simulink library "SkywardBLIMP_back"  (R2015a)
settings: Solver=ode45  StartTime=0.0  StopTime=10.0  RelTol=1e-3
settings Model: Creator=Francescodario  LastModifiedBy=franc

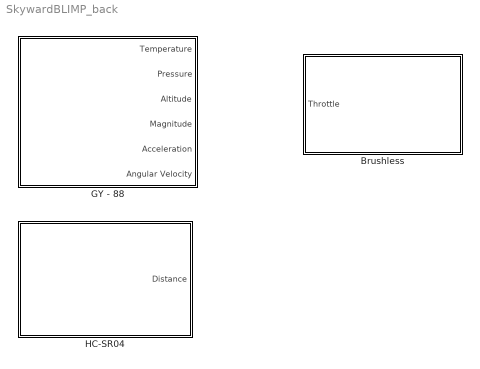
== system SkywardBLIMP_back ==
  Brushless : Subsystem  mask{PIN=9, S_T=0.01}
      mask prompts: S_T "Sample Time"
      mask help:
      | This block drive the Brushless motors of the BLIMP. Please do not modify the internal subsystem
      | parameters.
      mask Display:
      | %Load the image
      | rgb = imread('blocks\ESC\ESC.jpg');
      | % Display the image
      | image(rgb);
      | port_label('input',1,'Throttle')
  "GY - 88 " : Subsystem  mask(GY-88){S_T=0.02}
      mask prompts: S_T "Sample Time"
      mask help:
      | This block will output data from GY-88 IMU. Magnitude, Acceleration and Angular Velocity are
      | given as 3 components vectors.
      mask Display:
      | %Load the image
      | rgb = imread('blocks\GY-88\GY-88.jpg');
      | % Display the image
      | image(rgb);
      | %Port labels
      | port_label('output',1,'Temperature')
      | port_label('output',2,'Pressure')
      | port_label('output',3,'Altitude')
      | port_label('output',4,'Magnitude')
      | port_label('output',5,'Acceleration')
      | port_label('output',6,'Angular Velocity')
  HC-SR04 : Subsystem  mask{S_T=0.02}
      mask prompts: S_T "Sample Time"
      mask help:
      | This block drive the HC-SR04 ultrasonic sensor.
      | The Trig PIN should be connected to Arduino PIN 3, the Echo PIN should be
      | connected to Arduino PIN 2.
      mask Display:
      | %Load the image
      | rgb = imread('blocks\HC-SR04\HC-SR04.jpg');
      | % Display the image
      | image(rgb);
      | port_label('output',1,'Distance')

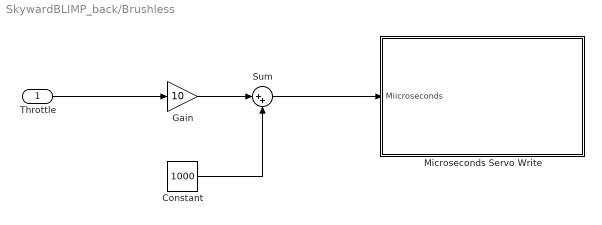
== system SkywardBLIMP_back/Brushless ==
  Throttle : Inport
  Constant : Constant  Value=1000
  Gain : Gain  Gain=10
  Microseconds Servo Write : Subsystem  mask{S_T=S_T, PIN=PIN}
      mask prompts: S_T "Sample Time"
  Sum : Sum  Inputs=|++
  wires:
  Constant/1 -> Sum/2
  Sum/1 -> Microseconds Servo Write/1("Miicroseconds ")
  Throttle/1 -> Gain/1
  Gain/1 -> Sum/1

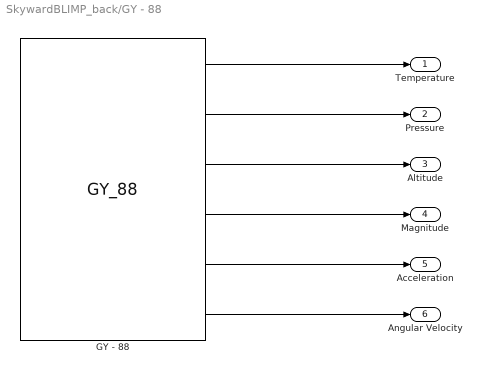
== system SkywardBLIMP_back/GY - 88  ==
  "GY - 88 " : S-Function  InitFcn=try, set_param(gcb,'FunctionName','GY_88'), end  FunctionName=GY_88  Parameters=0.02  SFunctionModules=GY_88_wrapper  mask(S-Function Builder){}
      mask help: Simulink:masks:SFunctionBuilder_MD
      mask init:
      | val = [[.9  0.75 0.75 1 1 .9 .9 1]',[1 1 0.75 0.75 .9 .9 1 .9]'];try , sys = get_param(gcb,'SfunBuilderFcnName');if isempty(sys), sys = get_param(gcb,'FunctionName'); end,catch, sys = get_param(gcb,'FunctionName'); end
      settings: CopyFcn=set_param(gcbh,'LinkStatus','none')  PreSaveFcn=try, set_param(gcb,'FunctionName','GY_88'), end  OpenFcn=sfunctionwizard(gcbh)
      mask Display: plot(val(:,1),val(:,2)),disp(sys), port_label('output',1,'temperature'), port_label('output',2,'pressure'), port_label('output',3,'altitude'), port_label('output',4,'magnitude'), port_label('output',5,'acceleration'), port_label('output',6,'angular_velocity')
  Temperature : Outport
  Pressure : Outport  Port=2
  Altitude : Outport  Port=3
  Magnitude : Outport  Port=4
  Acceleration : Outport  Port=5
  Angular Velocity : Outport  Port=6
  wires:
  "GY - 88 "/5 -> Acceleration/1
  "GY - 88 "/3 -> Altitude/1
  "GY - 88 "/6 -> Angular Velocity/1
  "GY - 88 "/2 -> Pressure/1
  "GY - 88 "/4 -> Magnitude/1
  "GY - 88 "/1 -> Temperature/1

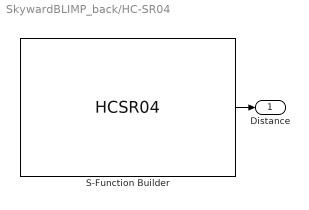
== system SkywardBLIMP_back/HC-SR04 ==
  S-Function Builder : S-Function  InitFcn=try, set_param(gcb,'FunctionName','HCSR04'), end  FunctionName=HCSR04  Parameters=0.01  SFunctionModules=HCSR04_wrapper  mask(S-Function Builder){}
      mask help: Simulink:masks:SFunctionBuilder_MD
      mask init: same as SkywardBLIMP_back/GY - 88 /GY - 88 
      settings: CopyFcn=set_param(gcbh,'LinkStatus','none')  PreSaveFcn=try, set_param(gcb,'FunctionName','HCSR04'), end  OpenFcn=sfunctionwizard(gcbh)
      mask Display: plot(val(:,1),val(:,2)),disp(sys), port_label('output',1,'distance')
  "Distance " : Outport
  wires:
  S-Function Builder/1 -> "Distance "/1

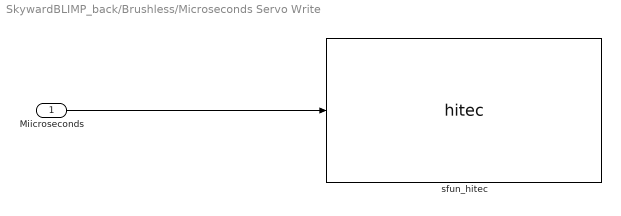
== system SkywardBLIMP_back/Brushless/Microseconds Servo Write ==
  "Miicroseconds " : Inport
  "sfun_hitec " : S-Function  InitFcn=try, set_param(gcb,'FunctionName','hitec'), end  FunctionName=hitec  Parameters=0.01,9  SFunctionModules=hitec_wrapper  mask(S-Function Builder){}
      mask help: Simulink:masks:SFunctionBuilder_MD
      mask init: same as SkywardBLIMP_back/GY - 88 /GY - 88 
      settings: CopyFcn=set_param(gcbh,'LinkStatus','none')  PreSaveFcn=try, set_param(gcb,'FunctionName','hitec'), end  OpenFcn=sfunctionwizard(gcbh)
      mask Display: plot(val(:,1),val(:,2)),disp(sys), port_label('input',1,'micros')
  wires:
  "Miicroseconds "/1 -> "sfun_hitec "/1
